simulink model "linear_interpolation"  (R2020b)
settings: Solver=FixedStepAuto  StartTime=0.0  StopTime=10.0  RelTol=1e-3
settings Model: Creator=conno  LastModifiedBy=conno

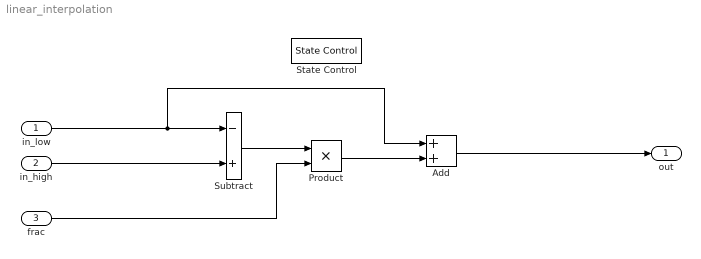
== system linear_interpolation ==
  in_low : Inport  OutDataTypeStr=gain_coeff_type
  in_high : Inport  Port=2  OutDataTypeStr=gain_coeff_type
  frac : Inport  Port=3  OutDataTypeStr=frac_coeff_type
  Add : Sum
  Product : Product  OutDataTypeStr=Inherit: Same as first input
  State Control : StateControl  StateControl=Synchronous
  Subtract : Sum  Inputs=-+
  out : Outport
  wires:
  Add/1 -> out/1
  in_low/1 -> Add/1, Subtract/1
  Subtract/1 -> Product/1
  in_high/1 -> Subtract/2
  frac/1 -> Product/2
  Product/1 -> Add/2
